simulink library "PerfectSurveillanceBlock"  (R2018b)
settings: Solver=VariableStepAuto  StartTime=0.0  StopTime=10.0  RelTol=1e-3
libraries: CreateCovDiagMatrix x1
settings Model: Creator=BI28030  LastModifiedBy=BI28030

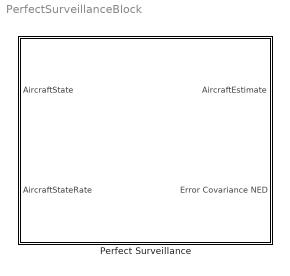
== system PerfectSurveillanceBlock ==
  Perfect Surveillance : Subsystem  Description=|  mask{dt=0.1}
      | Documentation for Perfect Observation Block                                                                                                                                                                                                                                                                                                                                                                                                          
      |                                                                                                                                                                                                                                                                                                                                                                                                                                                      
      | Description:  The perfect observation block, also known as a perfect                                                                                                                                                                                                                                                                                                                                                                                 
      | surveillance block, receives an Aircraft State, nominally from a Basic                                                                                                                                                                                                                                                                                                                                                                               
      | Aircraft Dynamics block, and outputs an Aircraft Estimate.  The Aircraft                                                                                                                                                                                                                                                                                                                                                                             
      | State that is received as input consists of Latitude, Longitude, and                                                                                                                                                                                                                                                                                                                                                                                 
      | Altitude state information as well as the aircraft position in local                                                                                                                                                                                                                                                                                                                                                                                 
      | coordinates in units of feet for north, east, and height.  The Aircraft                                                                                                                                                                                                                                                                                                                                                                              
      | Estimate outputs consist of estimates for the aircraft Latitude, Longitude, and Altitude, the east, north up position, and sensor covariance.  For perfect surveillance, the covariance estimates are all set to zero as default.  In addition, "time of validity" and a Boolean flag for the sensor report, "is Valid", are outputted as part of the Aircraft Estimate.                                                                             
      |                                                                                                                                                                                                                                                                                                                                                                                                                                                      
      | The initial perfect surveillance block developed receives the aircraft state information from the "AC2 - Basic Aircraft Dynamics" block within the "nominalEncounter" study.  Since the expected output from the AC1 and AC2 aircraft states have slightly different output parameters than what is provided from the perfect surveillance block (i.e., covariance estimates, isValid, and time of validity), the perfect surveillance block         
      | AircraftEstimate output has been left disconnected.                                                                                                                                                                                                                                                                                                                                                                                                  
      |                                                                                                                                                                                                                                                                                                                                                                                                                                                      
      | The initial unit test performed for this perfect observation block was to                                                                                                                                                                                                                                                                                                                                                                            
      | run the nominalEncounter study and to ensure that the simulation completes and no exceptions are encountered.  This unit test was successful (other than receiving a warning that the output of the perfect surveillance block is not connected, which was expected).  A more comprehensive future unit test would be to evaluate the position inputs and compare them with the position outputs to ensure that they are consistent with one another.
      mask prompts: dt "Dynamics Update Step Size (s)"

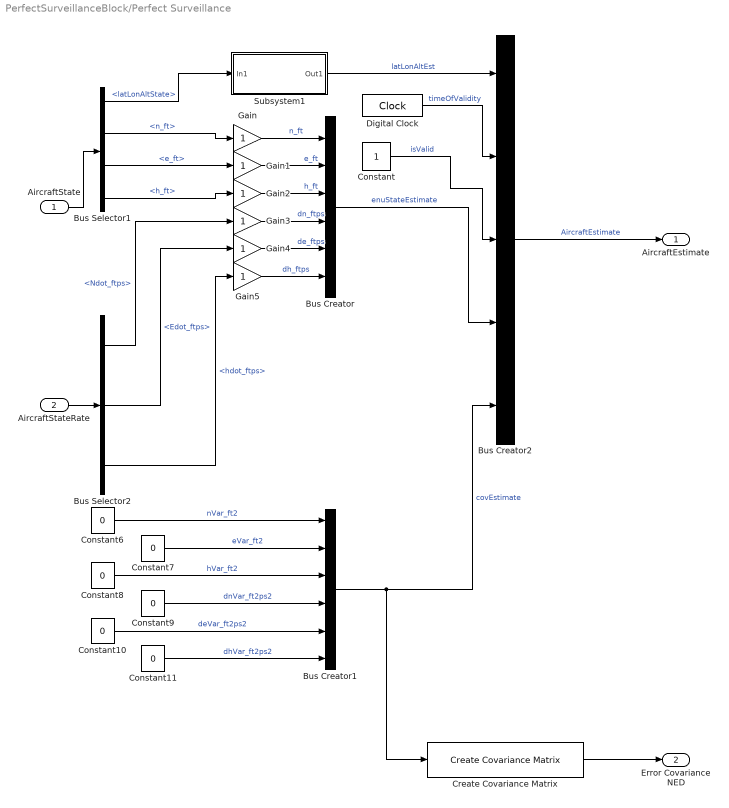
== system PerfectSurveillanceBlock/Perfect Surveillance ==
  AircraftState : Inport  OutDataTypeStr=Bus: AircraftState
  AircraftStateRate : Inport  Port=2  OutDataTypeStr=Bus: AircraftStateRate
  Bus Creator : BusCreator  Inputs=6  OutDataTypeStr=Bus: StateEstimate
  Bus Creator1 : BusCreator  Inputs=6  OutDataTypeStr=Bus: CovarianceEstimate
  Bus Creator2 : BusCreator  Inputs=5  OutDataTypeStr=Bus: AircraftEstimate  NonVirtualBus=on
  Bus Selector1 : BusSelector  OutputSignals=latLonAltState,n_ft,e_ft,h_ft
  Bus Selector2 : BusSelector  OutputSignals=Ndot_ftps,Edot_ftps,hdot_ftps
  Constant : Constant  OutDataTypeStr=boolean
  Constant{6..11} (6 alike) : Constant  Value=0
  Create Covariance Matrix : CreateCovDiagMatrix/Create Covariance Matrix  SystemSampleTime=-1
  Digital Clock : DigitalClock  SampleTime=dt
  Gain{,1..5} (6 alike) : Gain
  Subsystem1 : Subsystem
  AircraftEstimate : Outport  OutDataTypeStr=Bus: AircraftEstimate
  Error Covariance NED : Outport  Port=2
  wires:
  Gain5/1 -> Bus Creator/6  "dh_ftps"
  Gain4/1 -> Bus Creator/5  "de_ftps"
  Gain3/1 -> Bus Creator/4  "dn_ftps"
  Gain2/1 -> Bus Creator/3  "h_ft"
  Gain1/1 -> Bus Creator/2  "e_ft"
  Gain/1 -> Bus Creator/1  "n_ft"
  AircraftStateRate/1 -> Bus Selector2/1
  Subsystem1/1(Out1) -> Bus Creator2/1  "latLonAltEst"
  Digital Clock/1 -> Bus Creator2/2  "timeOfValidity"
  Constant/1 -> Bus Creator2/3  "isValid"
  Bus Selector1/1 -> Subsystem1/1(In1)  "<latLonAltState>"
  Bus Selector2/3 -> Gain5/1  "<hdot_ftps>"
  Bus Selector2/2 -> Gain4/1  "<Edot_ftps>"
  Bus Selector2/1 -> Gain3/1  "<Ndot_ftps>"
  Bus Selector1/4 -> Gain2/1  "<h_ft>"
  Bus Selector1/3 -> Gain1/1  "<e_ft>"
  Bus Selector1/2 -> Gain/1  "<n_ft>"
  AircraftState/1 -> Bus Selector1/1
  Constant11/1 -> Bus Creator1/6  "dhVar_ft2ps2"
  Constant10/1 -> Bus Creator1/5  "deVar_ft2ps2"
  Constant9/1 -> Bus Creator1/4  "dnVar_ft2ps2"
  Constant8/1 -> Bus Creator1/3  "hVar_ft2"
  Constant7/1 -> Bus Creator1/2  "eVar_ft2"
  Constant6/1 -> Bus Creator1/1  "nVar_ft2"
  Bus Creator2/1 -> AircraftEstimate/1  "AircraftEstimate"
  Bus Creator1/1 -> Create Covariance Matrix/1, Bus Creator2/5  "covEstimate"
  Bus Creator/1 -> Bus Creator2/4  "enuStateEstimate"
  Create Covariance Matrix/1 -> Error Covariance NED/1

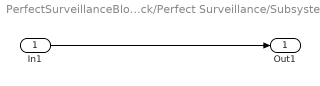
== system PerfectSurveillanceBlock/Perfect Surveillance/Subsystem1 ==
  In1 : Inport
  Out1 : Outport
  wires:
  In1/1 -> Out1/1
